simulink library "gs_estimation_lib"  (R2016b)
settings: Solver=ode45  StartTime=0.0  StopTime=86400  RelTol=1e-3  EnableMultiTasking=on
settings Model: Creator=Taylor  LastModifiedBy=Sean
settings DataIOCC: LimitDataPoints=on
settings OptimizationCC: LifeSpan=inf
settings DebuggingCC: AllowSymbolicDim=off  SFUnexpectedBacktrackingDiag=warning  SFNoUnconditionalDefaultTransitionDiag=warning  SFExecutionAtInitializationDiag=none
settings GRTTargetCC: TargetLangStandard=C89/C90 (ANSI)  GeneratePreprocessorConditionals=Disable all
settings ConfigComp: CovMetricSettings=dw  CovHtmlReporting=on  CovSaveCumulativeToWorkspaceVar=on  CovSaveSingleToWorkspaceVar=on  CovExternalEMLEnable=off

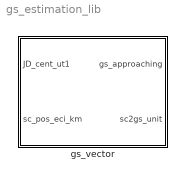
== system gs_estimation_lib ==
  gs_vector : Subsystem

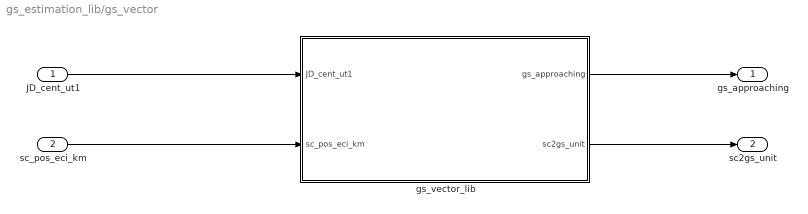
== system gs_estimation_lib/gs_vector ==
  JD_cent_ut1 : Inport
  sc_pos_eci_km : Inport  Port=2
  gs_vector_lib : Subsystem
  gs_approaching : Outport
  sc2gs_unit : Outport  Port=2
  wires:
  JD_cent_ut1/1 -> gs_vector_lib/1(JD_cent_ut1)
  gs_vector_lib/1(gs_approaching) -> gs_approaching/1
  sc_pos_eci_km/1 -> gs_vector_lib/2(sc_pos_eci_km)
  gs_vector_lib/2(sc2gs_unit) -> sc2gs_unit/1

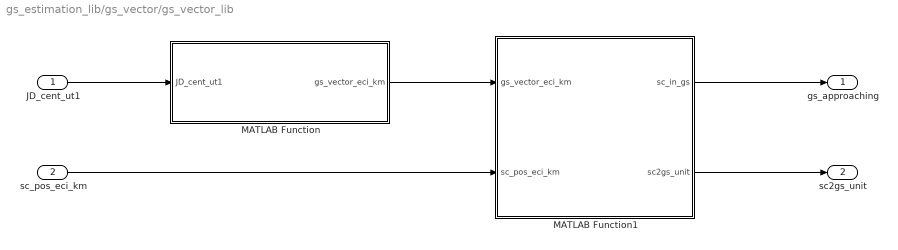
== system gs_estimation_lib/gs_vector/gs_vector_lib ==
  JD_cent_ut1 : Inport
  sc_pos_eci_km : Inport  Port=2
  MATLAB Function : MATLAB Function  TreatAsAtomicUnit=on
  MATLAB Function1 : MATLAB Function  TreatAsAtomicUnit=on
  gs_approaching : Outport
  sc2gs_unit : Outport  Port=2
  wires:
  JD_cent_ut1/1 -> MATLAB Function/1(JD_cent_ut1)
  MATLAB Function/1(gs_vector_eci_km) -> MATLAB Function1/1(gs_vector_eci_km)
  sc_pos_eci_km/1 -> MATLAB Function1/2(sc_pos_eci_km)
  MATLAB Function1/2(sc2gs_unit) -> sc2gs_unit/1
  MATLAB Function1/1(sc_in_gs) -> gs_approaching/1

== matlab function gs_estimation_lib/gs_vector/gs_vector_lib/MATLAB Function1 ==
  data: gs_vector_eci_km input; sc_in_gs output; sc2gs_unit output; sc_pos_eci_km input
function [sc_in_gs,sc2gs_unit] = sc_approaching_gs(gs_vector_eci_km,sc_pos_eci_km)

% Constants
M2KM        = 1000;
ECCE2       = 0.006694385000;
RE          = 6378.137;
TRUE        = 1;
FALSE       = 0;
% -----

% Main Function
LOS     = FALSE;

gs_vector_eci_km(3)    = gs_vector_eci_km(3)/(sqrt(1 - ECCE2));
sc_pos_eci_km(3)        = sc_pos_eci_km(3)/(sqrt(1 - ECCE2));

gs_vec     = gs_vector_eci_km;
sc_vec      = sc_pos_eci_km;

sc2gs_unit  = (gs_vec - sc_vec)/norm(gs_vec - sc_vec);

% Determine if the sc is in the light or shadow
%   Call vector 1 the gs, vector 2 the sc

mag1    = norm(gs_vec);
mag2    = norm(sc_vec);

mag1_sq     = mag1*mag1;
mag2_sq     = mag2*mag2;

gs_sc_dot  = dot(gs_vec,sc_vec);

% Find t_min
t_min_num   = mag1_sq - gs_sc_dot;
t_min_den   = mag1_sq + mag2_sq - 2*gs_sc_dot;

if ( t_min_den < 0.0001  )
    t_min= 0.0;
else
    t_min = ( t_min_num ) / ( t_min_den );
end

c_t_min_sq  = ((1-t_min)*mag1_sq + gs_sc_dot*t_min)/RE^2;

% Check LoS
if t_min < 0 || t_min > 1
    LOS     = TRUE;
elseif c_t_min_sq >= 1
    LOS     = FALSE;
end

sc_in_gs   = LOS;

== matlab function gs_estimation_lib/gs_vector/gs_vector_lib/MATLAB Function ==
  data: JD_cent_ut1 input; gs_vector_eci_km output
function gs_vector_eci_km = gs_vector(JD_cent_ut1)

% Constants
AU2KM  = 149597870.700; 
DEG2RAD     = pi/180.0;
% -----

% Convert to Julian Centuries since J2000
% JD_cent_ut1     = (JD_ut1 - 2451545)/36525;

% Mean longitude in a mean-equator of date frame
mean_long_gs  = rem(280.460 + 36000.771*JD_cent_ut1,360); % [deg]

% Mean anomaly for the gs. Low precision formula since we're approximating
% T_TDB with T_UT1.
mean_anom_gs   = rem(357.5291092 + 35999.05034*JD_cent_ut1,360); %[deg]
mean_anom_gs_rad   = DEG2RAD*mean_anom_gs;

% Make sure we're \in [0,2pi]
if ( mean_anom_gs_rad < 0.0  )
    mean_anom_gs_rad = 2*pi + mean_anom_gs_rad;
end

% Approximate the ecliptic longitude of the gs
long_eclp       = mean_long_gs + 1.914666471*sin(mean_anom_gs_rad) + ...
                    0.019994643*sin(2*mean_anom_gs_rad); %[deg]
long_eclp_rad   = rem(DEG2RAD*long_eclp,360); % [rad]            
       
% Assume the ecliptic latitude is zero
lat_eclp     = 0; %[deg]

% Approximate the obliquity of the ecliptic using
oblq        = 23.439291 - 0.0130042*JD_cent_ut1;
oblq_rad    = DEG2RAD*oblq;

% Find the distance in AU from E to S
r           =  1.000140612 - 0.016708617*cos(mean_anom_gs_rad) - ...
                    0.000139589*cos(2*mean_anom_gs_rad);

x_MOD_km    = r*cos(long_eclp_rad)*AU2KM;
y_MOD_km    = r*cos(oblq_rad)*sin(long_eclp_rad)*AU2KM;
z_MOD_km    = r*sin(oblq_rad)*sin(long_eclp_rad)*AU2KM;

gs_vector_mod_km = [x_MOD_km; y_MOD_km; z_MOD_km];

% Convert to ECI (mean-equator-mean-equinox) frame 

gs_vector_eci_km   = mod2eci(gs_vector_mod_km,JD_cent_ut1);

end

function vec_eci = mod2eci(vec_mod,JD_cent_ut1)

[prec,psia,wa,ea,xa] = precess ( JD_cent_ut1 );

vec_eci = prec*vec_mod;

end

function [prec,psia,wa,ea,xa] = precess ( ttt )

        
        % " to rad
        convrt = pi / (180.0*3600.0);

          % ------------------ iau 03 precession angles -------------------
            oblo =  84381.406; % "
            psia =  (((( -0.0000000951 * ttt + 0.000132851 ) * ttt - 0.00114045 ) * ttt - 1.0790069 ) * ttt + 5038.481507 ) * ttt; % "
            wa   =  ((((  0.0000003337 * ttt - 0.000000467 ) * ttt - 0.00772503 ) * ttt + 0.0512623 ) * ttt -    0.025754 ) * ttt + oblo;
            ea   =  (((( -0.0000000434 * ttt - 0.000000576 ) * ttt + 0.00200340 ) * ttt - 0.0001831 ) * ttt -   46.836769 ) * ttt + oblo;
            xa   =  (((( - 0.0000000560 * ttt + 0.000170663 ) * ttt - 0.00121197 ) * ttt - 2.3814292 ) * ttt +   10.556403 ) * ttt;

            zeta =  (((( - 0.0000003173 * ttt - 0.000005971 ) * ttt + 0.01801828 ) * ttt + 0.2988499 ) * ttt + 2306.083227 ) * ttt + 2.650545; % "
            theta=  (((( - 0.0000001274 * ttt - 0.000007089 ) * ttt - 0.04182264 ) * ttt - 0.4294934 ) * ttt + 2004.191903 ) * ttt;
            z    =  ((((   0.0000002904 * ttt - 0.000028596 ) * ttt + 0.01826837 ) * ttt + 1.0927348 ) * ttt + 2306.077181 ) * ttt - 2.650545;
        
        % convert all units to rad
        psia = psia  * convrt; % rad
        wa   = wa    * convrt;
        ea   = ea    * convrt;
        xa   = xa    * convrt;

            oblo = oblo * convrt; % " to rad
            a4  = rot3mat(-xa);
            a5  = rot1mat(wa);
            a6  = rot3mat(psia);
            a7  = rot1mat(-oblo);
            prec = a7*a6*a5*a4;
        
end % precess

function DCMx = rot1mat(x_rad)

s   = sin( x_rad );
c   = cos( x_rad );

DCMx    = [ 1   0   0
            0   c   s;
            0  -s   c ];

end

function DCMz   = rot3mat(z_rad)

s   = sin( z_rad );
c   = cos( z_rad );

DCMz    = [ c   s   0;
           -s   c   0;
            0   0   1 ];

end
